simulink library "myLib_R2020a"  (R2020a)
settings: Solver=VariableStepAuto  StartTime=0.0  StopTime=10.0  RelTol=1e-3
libraries: $bdroot x26, simulink x10
settings Model: Creator=Administrator  LastModifiedBy=Administrator

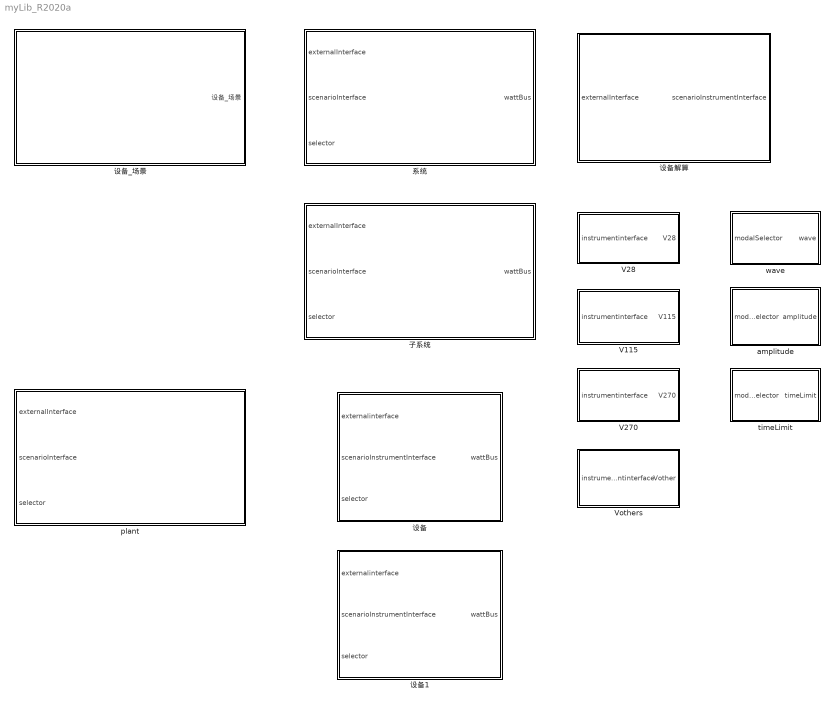
== system myLib_R2020a ==
  V115 : Subsystem  mask{V115_amplitudeData=0, V115_waveData=0, V115_timeLimitData=0}
      settings: CopyFcn=set_param(gcbh,'LinkStatus','none');
  V270 : Subsystem  mask{V270_amplitudeData=0, V270_waveData=0, V270_timeLimitData=0}
      settings: CopyFcn=set_param(gcbh,'LinkStatus','none');
  V28 : Subsystem  mask{V28_amplitudeData=0, V28_waveData=0, V28_timeLimitData=0}
      settings: CopyFcn=set_param(gcbh,'LinkStatus','none');
  Vothers : Subsystem  mask{Vother_amplitudeData=0, Vother_waveData=0, Vother_timeLimitData=0}
      settings: CopyFcn=set_param(gcbh,'LinkStatus','none');
  amplitude : Subsystem  mask{amplitudeData=[5,6,4,9,2,10]}
      settings: CopyFcn=set_param(gcbh,'LinkStatus','none');
  plant : Subsystem
      settings: CopyFcn=set_param(gcbh,'LinkStatus','none');
  timeLimit : Subsystem  mask{timeLimitData=[1 2 3 4 5 6]}
      settings: CopyFcn=set_param(gcbh,'LinkStatus','none');
  wave : Subsystem  mask{waveData=[1,2;3,4;5,6;7,8;1,2;3,4;5,6;7,8]'}
      settings: CopyFcn=set_param(gcbh,'LinkStatus','none');
      mask DialogControl ParameterGroupVar Prompt: 说明
  子系统 : Subsystem
      settings: CopyFcn=set_param(gcbh,'LinkStatus','none');
  系统 : Subsystem
      settings: CopyFcn=set_param(gcbh,'LinkStatus','none');
  设备 : Subsystem
      settings: CopyFcn=set_param(gcbh,'LinkStatus','none');
  设备1 : Subsystem
      settings: CopyFcn=set_param(gcbh,'LinkStatus','none');
  设备_场景 : Subsystem  mask{modalSelectorSig=[0 1;0 0;1 2;1 2;0 0], triggerSig=[0 1;0 0;1 0;1 0;0 0], sampleTime=-1}
      mask prompts: modalSelectorSig "模态选择信号"; triggerSig "触发信号"; sampleTime "采样时间"
  设备解算 : Subsystem

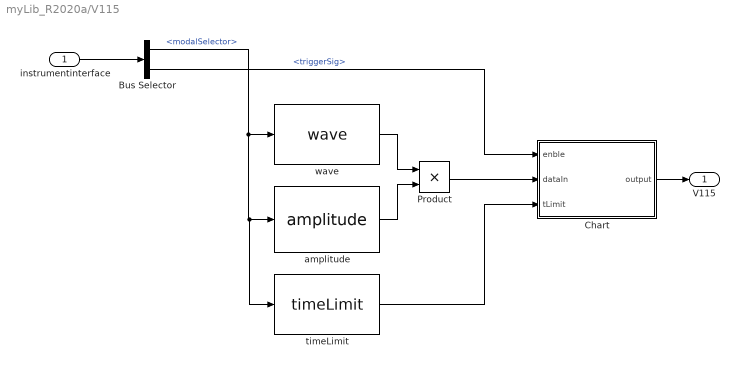
== system myLib_R2020a/V115 ==
  instrumentinterface : Inport  OutDataTypeStr=Bus: instrumentBus
  Bus Selector : BusSelector  OutputSignals=modalSelector,triggerSig
  Chart : Stateflow chart  TreatAsAtomicUnit=on
  Product : Product
  amplitude : $bdroot/amplitude  amplitudeData=V115_amplitudeData
  timeLimit : $bdroot/timeLimit  timeLimitData=V115_timeLimitData
  wave : $bdroot/wave  waveData=V115_waveData
  V115 : Outport
  wires:
  Chart/1(output) -> V115/1
  Bus Selector/1 -> wave/1, amplitude/1, timeLimit/1  "<modalSelector>"
  wave/1 -> Product/1
  Product/1 -> Chart/2(dataIn)
  amplitude/1 -> Product/2
  instrumentinterface/1 -> Bus Selector/1
  Bus Selector/2 -> Chart/1(enble)  "<triggerSig>"
  timeLimit/1 -> Chart/3(tLimit)

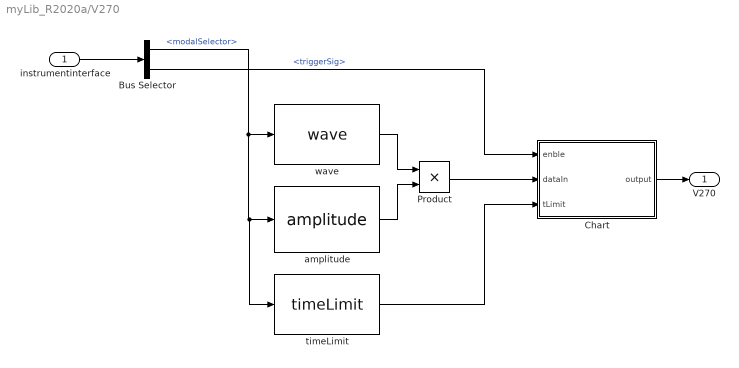
== system myLib_R2020a/V270 ==
  instrumentinterface : Inport  OutDataTypeStr=Bus: instrumentBus
  Bus Selector : BusSelector  OutputSignals=modalSelector,triggerSig
  Chart : Stateflow chart  TreatAsAtomicUnit=on
  Product : Product
  amplitude : $bdroot/amplitude  amplitudeData=V270_amplitudeData
  timeLimit : $bdroot/timeLimit  timeLimitData=V270_timeLimitData
  wave : $bdroot/wave  waveData=V270_waveData
  V270 : Outport
  wires:
  Chart/1(output) -> V270/1
  Bus Selector/1 -> timeLimit/1, amplitude/1, wave/1  "<modalSelector>"
  wave/1 -> Product/1
  Product/1 -> Chart/2(dataIn)
  amplitude/1 -> Product/2
  instrumentinterface/1 -> Bus Selector/1
  Bus Selector/2 -> Chart/1(enble)  "<triggerSig>"
  timeLimit/1 -> Chart/3(tLimit)

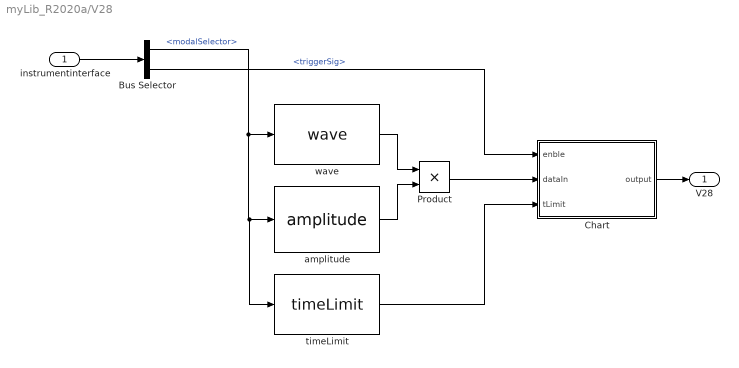
== system myLib_R2020a/V28 ==
  instrumentinterface : Inport  OutDataTypeStr=Bus: instrumentBus
  Bus Selector : BusSelector  OutputSignals=modalSelector,triggerSig
  Chart : Stateflow chart  TreatAsAtomicUnit=on
  Product : Product
  amplitude : $bdroot/amplitude  amplitudeData=V28_amplitudeData
  timeLimit : $bdroot/timeLimit  timeLimitData=V28_timeLimitData
  wave : $bdroot/wave  waveData=V28_waveData
  V28 : Outport
  wires:
  instrumentinterface/1 -> Bus Selector/1
  Bus Selector/1 -> wave/1, timeLimit/1, amplitude/1  "<modalSelector>"
  Bus Selector/2 -> Chart/1(enble)  "<triggerSig>"
  timeLimit/1 -> Chart/3(tLimit)
  wave/1 -> Product/1
  amplitude/1 -> Product/2
  Product/1 -> Chart/2(dataIn)
  Chart/1(output) -> V28/1

== system myLib_R2020a/Vothers ==
  instrumentinterface : Inport  OutDataTypeStr=Bus: instrumentBus
  Bus Selector : BusSelector  OutputSignals=modalSelector,triggerSig
  Chart : Stateflow chart  TreatAsAtomicUnit=on
  Product : Product
  amplitude : $bdroot/amplitude  amplitudeData=Vother_amplitudeData
  timeLimit : $bdroot/timeLimit  timeLimitData=Vother_timeLimitData
  wave : $bdroot/wave  waveData=Vother_waveData
  Vother : Outport
  wires:
  Chart/1(output) -> Vother/1
  Bus Selector/1 -> wave/1, amplitude/1, timeLimit/1  "<modalSelector>"
  wave/1 -> Product/1
  Product/1 -> Chart/2(dataIn)
  amplitude/1 -> Product/2
  instrumentinterface/1 -> Bus Selector/1
  Bus Selector/2 -> Chart/1(enble)  "<triggerSig>"
  timeLimit/1 -> Chart/3(tLimit)

== system myLib_R2020a/amplitude ==
  modalSelector : Inport
  Selector : Selector  IndexOptions=Starting index (port)  Indices=[1 3]  OutputSizes=1
  amplitudes : Constant  Value=amplitudeData
  amplitude : Outport
  wires:
  amplitudes/1 -> Selector/1
  modalSelector/1 -> Selector/2
  Selector/1 -> amplitude/1

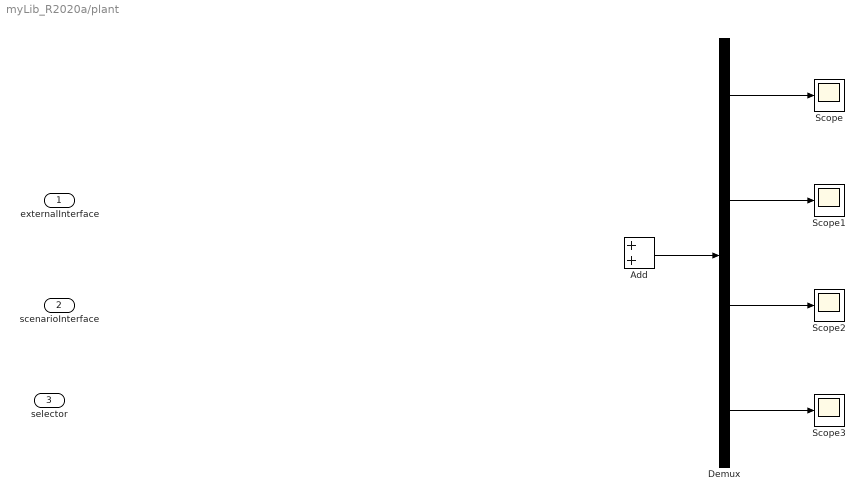
== system myLib_R2020a/plant ==
  externalInterface : Inport  OutDataTypeStr=Bus: externalBus
  scenarioInterface : Inport  Port=2  OutDataTypeStr=Bus: scenarioInstrumentBus
  selector : Inport  Port=3
  Add : Sum
  Demux : Demux
  Scope{,1..3} (4 alike) : Scope
      Scope1 settings: CopyFcn=set_param(gcbh,'LinkStatus','none');
  wires:
  Add/1 -> Demux/1
  Demux/1 -> Scope/1
  Demux/2 -> Scope1/1
  Demux/3 -> Scope2/1
  Demux/4 -> Scope3/1

== system myLib_R2020a/timeLimit ==
  modalSelector : Inport
  Selector1 : Selector  IndexOptions=Starting index (port)  Indices=[1 3]  OutputSizes=1
  timeLimits : Constant  Value=timeLimitData
  timeLimit : Outport
  wires:
  modalSelector/1 -> Selector1/2
  Selector1/1 -> timeLimit/1
  timeLimits/1 -> Selector1/1

== system myLib_R2020a/wave ==
  modalSelector : Inport
  Constant1 : Constant  Value=waveData
  Direct Lookup Table (n-D) : LookupNDDirect  InputsSelectThisObjectFromTable=Vector  TableIsInput=on  Table=[4 5 6;16 19 20;10 18 23]'
  Display : Display
  wave : Outport
  wires:
  Direct Lookup Table (n-D)/1 -> wave/1, Display/1
  Constant1/1 -> Direct Lookup Table (n-D)/2
  modalSelector/1 -> Direct Lookup Table (n-D)/1

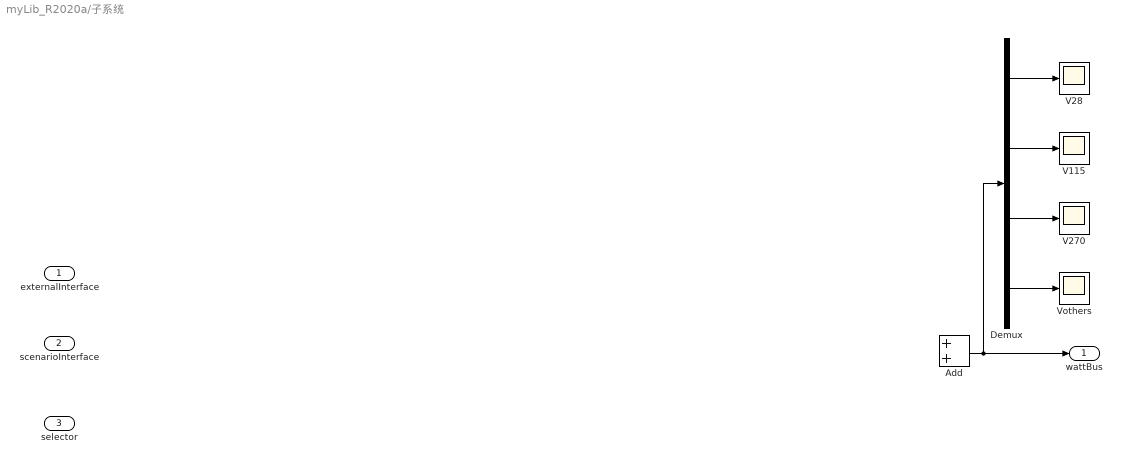
== system myLib_R2020a/子系统 ==
  externalInterface : Inport  OutDataTypeStr=Bus: externalBus
  scenarioInterface : Inport  Port=2  OutDataTypeStr=Bus: scenarioBus
  selector : Inport  Port=3
  Add : Sum
  Demux : Demux
  V115 : Scope
      settings: LoadFcn=bl = gcb
  V270 : Scope
      settings: LoadFcn=bl = gcb
  V28 : Scope
      settings: LoadFcn=bl = gcb
  Vothers : Scope
      settings: LoadFcn=bl = gcb
  wattBus : Outport  OutDataTypeStr=Bus: wattBus
  wires:
  Add/1 -> Demux/1, wattBus/1
  Demux/1 -> V28/1
  Demux/2 -> V115/1
  Demux/3 -> V270/1
  Demux/4 -> Vothers/1

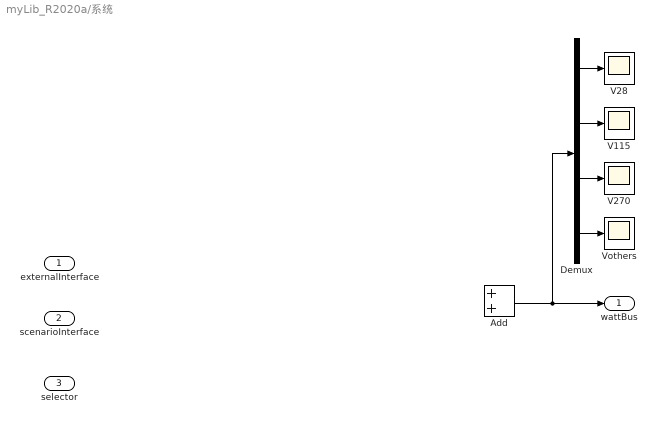
== system myLib_R2020a/系统 ==
  externalInterface : Inport  OutDataTypeStr=Bus: externalBus
  scenarioInterface : Inport  Port=2  OutDataTypeStr=Bus: scenarioBus
  selector : Inport  Port=3
  Add : Sum
  Demux : Demux
  V115 : Scope
  V270 : Scope
  V28 : Scope
  Vothers : Scope
  wattBus : Outport  OutDataTypeStr=Bus: wattBus
  wires:
  Add/1 -> Demux/1, wattBus/1
  Demux/1 -> V28/1
  Demux/2 -> V115/1
  Demux/3 -> V270/1
  Demux/4 -> Vothers/1

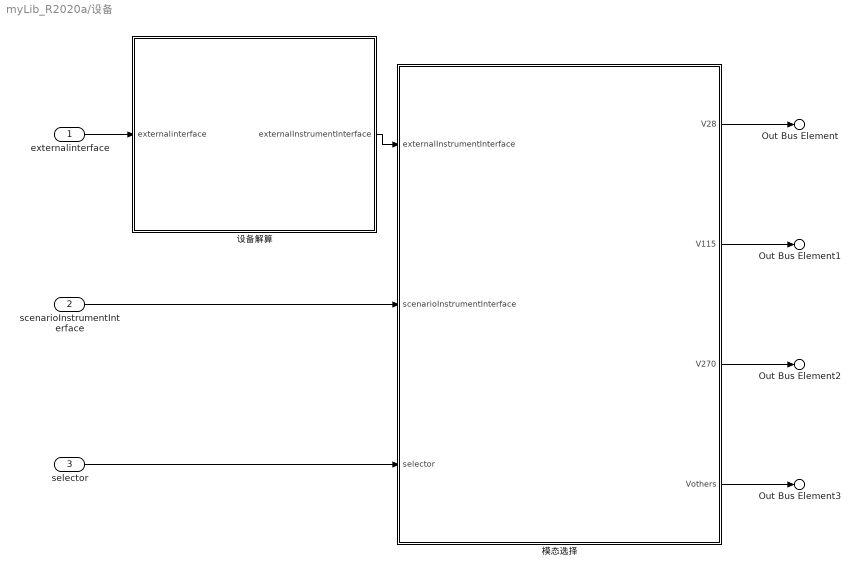
== system myLib_R2020a/设备 ==
  externalinterface : Inport  OutDataTypeStr=Bus: externalBus
  scenarioInstrumentInterface : Inport  Port=2  OutDataTypeStr=Bus: scenarioInstrumentBus
  selector : Inport  Port=3
  模态选择 : Subsystem
  设备解算 : Subsystem
  Out Bus Element : Outport  PortName=wattBus  Element=V28
  Out Bus Element1 : Outport  PortName=wattBus  Element=V115
  Out Bus Element2 : Outport  PortName=wattBus  Element=V270
  Out Bus Element3 : Outport  PortName=wattBus  Element=Vother
  wires:
  externalinterface/1 -> 设备解算/1(externalinterface)
  设备解算/1(externalInstrumentInterface) -> 模态选择/1(externalInstrumentInterface)
  scenarioInstrumentInterface/1 -> 模态选择/2(scenarioInstrumentInterface)
  模态选择/1(V28) -> Out Bus Element/1
  模态选择/2(V115) -> Out Bus Element1/1
  模态选择/3(V270) -> Out Bus Element2/1
  模态选择/4(Vothers) -> Out Bus Element3/1
  selector/1 -> 模态选择/3(selector)

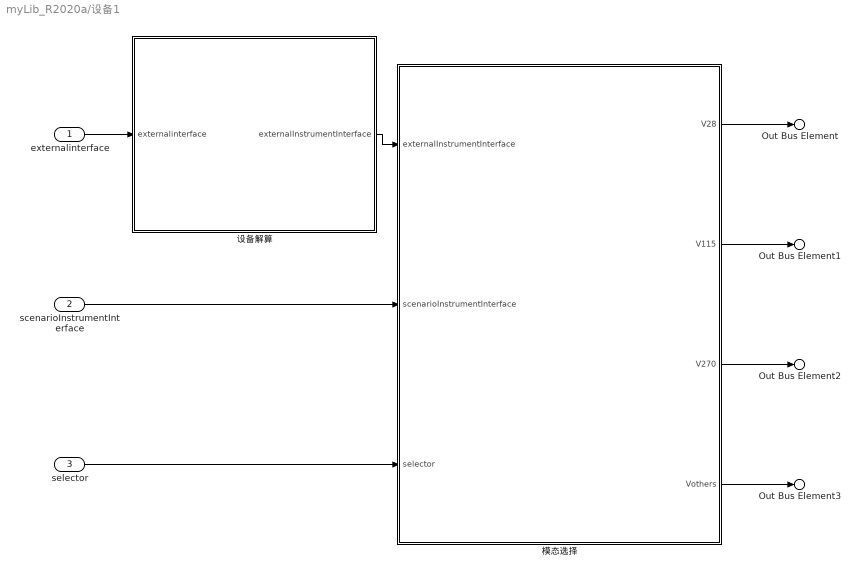
== system myLib_R2020a/设备1 ==
  externalinterface : Inport  OutDataTypeStr=Bus: externalBus
  scenarioInstrumentInterface : Inport  Port=2  OutDataTypeStr=Bus: scenarioInstrumentBus
  selector : Inport  Port=3
  模态选择 : Subsystem
  设备解算 : Subsystem
  Out Bus Element : Outport  PortName=wattBus  Element=V28
  Out Bus Element1 : Outport  PortName=wattBus  Element=V115
  Out Bus Element2 : Outport  PortName=wattBus  Element=V270
  Out Bus Element3 : Outport  PortName=wattBus  Element=Vother
  wires:
  externalinterface/1 -> 设备解算/1(externalinterface)
  设备解算/1(externalInstrumentInterface) -> 模态选择/1(externalInstrumentInterface)
  scenarioInstrumentInterface/1 -> 模态选择/2(scenarioInstrumentInterface)
  模态选择/1(V28) -> Out Bus Element/1
  模态选择/2(V115) -> Out Bus Element1/1
  模态选择/3(V270) -> Out Bus Element2/1
  模态选择/4(Vothers) -> Out Bus Element3/1
  selector/1 -> 模态选择/3(selector)

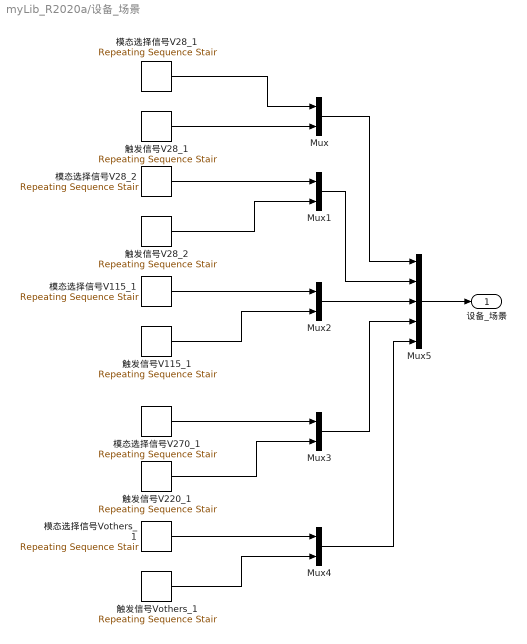
== system myLib_R2020a/设备_场景 ==
  Mux{,1..4} (5 alike) : Mux  Inputs=2
  Mux5 : Mux  Inputs=5
  模态选择信号V115_1 : simulink/Sources/Repeating Sequence Stair  OutValues=modalSelectorSig(3,:)  tsamp=sampleTime  OutMin=[]  OutMax=[]  OutDataTypeStr=double  OutputDataTypeScalingMode=double  OutDataType=fixdt(0,8)  ConRadixGroup=Best Precision: Vector-wise  OutScaling=2^-12
  模态选择信号V270_1 : simulink/Sources/Repeating Sequence Stair  OutValues=modalSelectorSig(4,:)  tsamp=sampleTime  OutMin=[]  OutMax=[]  OutDataTypeStr=double  OutputDataTypeScalingMode=double  OutDataType=fixdt(0,8)  ConRadixGroup=Best Precision: Vector-wise  OutScaling=2^-12
  模态选择信号V28_1 : simulink/Sources/Repeating Sequence Stair  OutValues=modalSelectorSig(1,:)  tsamp=sampleTime  OutMin=[]  OutMax=[]  OutDataTypeStr=double  OutputDataTypeScalingMode=double  OutDataType=fixdt(0,8)  ConRadixGroup=Best Precision: Vector-wise  OutScaling=2^-12
  模态选择信号V28_2 : simulink/Sources/Repeating Sequence Stair  OutValues=modalSelectorSig(2,:)  tsamp=sampleTime  OutMin=[]  OutMax=[]  OutDataTypeStr=double  OutputDataTypeScalingMode=double  OutDataType=fixdt(0,8)  ConRadixGroup=Best Precision: Vector-wise  OutScaling=2^-12
  模态选择信号Vothers_1 : simulink/Sources/Repeating Sequence Stair  OutValues=modalSelectorSig(5,:)  tsamp=sampleTime  OutMin=[]  OutMax=[]  OutDataTypeStr=double  OutputDataTypeScalingMode=double  OutDataType=fixdt(0,8)  ConRadixGroup=Best Precision: Vector-wise  OutScaling=2^-12
  触发信号V115_1 : simulink/Sources/Repeating Sequence Stair  OutValues=triggerSig(3,:)  tsamp=sampleTime  OutMin=[]  OutMax=[]  OutDataTypeStr=double  OutputDataTypeScalingMode=double  OutDataType=fixdt(0,8)  ConRadixGroup=Best Precision: Vector-wise  OutScaling=2^-12
  触发信号V220_1 : simulink/Sources/Repeating Sequence Stair  OutValues=triggerSig(4,:)  tsamp=sampleTime  OutMin=[]  OutMax=[]  OutDataTypeStr=double  OutputDataTypeScalingMode=double  OutDataType=fixdt(0,8)  ConRadixGroup=Best Precision: Vector-wise  OutScaling=2^-12
  触发信号V28_1 : simulink/Sources/Repeating Sequence Stair  OutValues=triggerSig(1,:)  tsamp=sampleTime  OutMin=[]  OutMax=[]  OutDataTypeStr=double  OutputDataTypeScalingMode=double  OutDataType=fixdt(0,8)  ConRadixGroup=Best Precision: Vector-wise  OutScaling=2^-12
  触发信号V28_2 : simulink/Sources/Repeating Sequence Stair  OutValues=triggerSig(2,:)  tsamp=sampleTime  OutMin=[]  OutMax=[]  OutDataTypeStr=double  OutputDataTypeScalingMode=double  OutDataType=fixdt(0,8)  ConRadixGroup=Best Precision: Vector-wise  OutScaling=2^-12
  触发信号Vothers_1 : simulink/Sources/Repeating Sequence Stair  OutValues=triggerSig(5,:)  tsamp=sampleTime  OutMin=[]  OutMax=[]  OutDataTypeStr=double  OutputDataTypeScalingMode=double  OutDataType=fixdt(0,8)  ConRadixGroup=Best Precision: Vector-wise  OutScaling=2^-12
  设备_场景 : Outport
  wires:
  模态选择信号V28_1/1 -> Mux/1
  触发信号V28_1/1 -> Mux/2
  模态选择信号V28_2/1 -> Mux1/1
  触发信号V28_2/1 -> Mux1/2
  模态选择信号V115_1/1 -> Mux2/1
  触发信号V115_1/1 -> Mux2/2
  模态选择信号V270_1/1 -> Mux3/1
  触发信号V220_1/1 -> Mux3/2
  模态选择信号Vothers_1/1 -> Mux4/1
  触发信号Vothers_1/1 -> Mux4/2
  Mux2/1 -> Mux5/3
  Mux/1 -> Mux5/1
  Mux1/1 -> Mux5/2
  Mux3/1 -> Mux5/4
  Mux4/1 -> Mux5/5
  Mux5/1 -> 设备_场景/1

== system myLib_R2020a/设备解算 ==
  externalInterface : Inport  OutDataTypeStr=Bus: externalBus
  scenarioInstrumentInterface : Outport  OutDataTypeStr=Bus: scenarioInstrumentBus

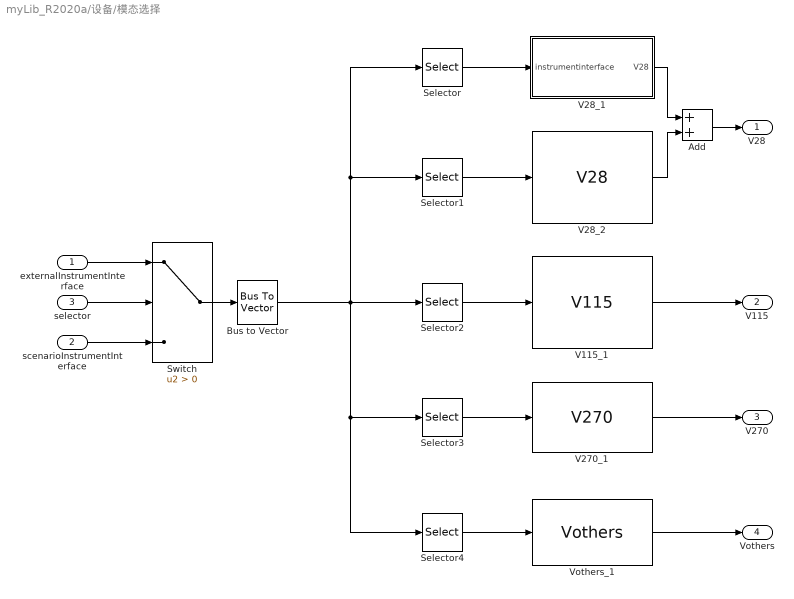
== system myLib_R2020a/设备/模态选择 ==
  externalInstrumentInterface : Inport  OutDataTypeStr=Bus: scenarioInstrumentBus
  scenarioInstrumentInterface : Inport  Port=2  OutDataTypeStr=Bus: scenarioBus
  selector : Inport  Port=3
  Add : Sum
  Bus to Vector : BusToVector
  Selector : Selector  InputPortWidth=10  IndexOptions=Index vector (dialog)  Indices=[1 6]  OutputSizes=1
  Selector1 : Selector  InputPortWidth=10  IndexOptions=Index vector (dialog)  Indices=[2 7]  OutputSizes=1
  Selector2 : Selector  InputPortWidth=10  IndexOptions=Index vector (dialog)  Indices=[3 8]  OutputSizes=1
  Selector3 : Selector  InputPortWidth=10  IndexOptions=Index vector (dialog)  Indices=[4 9]  OutputSizes=1
  Selector4 : Selector  InputPortWidth=10  IndexOptions=Index vector (dialog)  Indices=[5 10]  OutputSizes=1
  Switch : Switch  Criteria=u2 > Threshold
  V115_1 : $bdroot/V115  V115_amplitudeData=0  V115_waveData=0  V115_timeLimitData=0
  V270_1 : $bdroot/V270  V270_amplitudeData=0  V270_waveData=0  V270_timeLimitData=0
  V28_1 : Subsystem  mask{V28_amplitudeData=0, V28_waveData=0, V28_timeLimitData=0}
      settings: CopyFcn=set_param(gcbh,'LinkStatus','none');
  V28_2 : $bdroot/V28  V28_amplitudeData=0  V28_waveData=0  V28_timeLimitData=0
  Vothers_1 : $bdroot/Vothers  Vother_amplitudeData=0  Vother_waveData=0  Vother_timeLimitData=0
  V28 : Outport
  V115 : Outport  Port=2
  V270 : Outport  Port=3
  Vothers : Outport  Port=4
  wires:
  Selector1/1 -> V28_2/1
  Selector4/1 -> Vothers_1/1
  Selector2/1 -> V115_1/1
  Selector3/1 -> V270_1/1
  V270_1/1 -> V270/1
  V115_1/1 -> V115/1
  Vothers_1/1 -> Vothers/1
  selector/1 -> Switch/2
  externalInstrumentInterface/1 -> Switch/1
  scenarioInstrumentInterface/1 -> Switch/3
  Switch/1 -> Bus to Vector/1
  Selector/1 -> V28_1/1(instrumentinterface)
  Bus to Vector/1 -> Selector1/1, Selector/1, Selector4/1, Selector3/1, Selector2/1
  V28_1/1(V28) -> Add/1
  V28_2/1 -> Add/2
  Add/1 -> V28/1

== system myLib_R2020a/设备/设备解算 ==
  externalinterface : Inport  OutDataTypeStr=Bus: externalBus
  externalInstrumentInterface : Outport  OutDataTypeStr=Bus: scenarioInstrumentBus

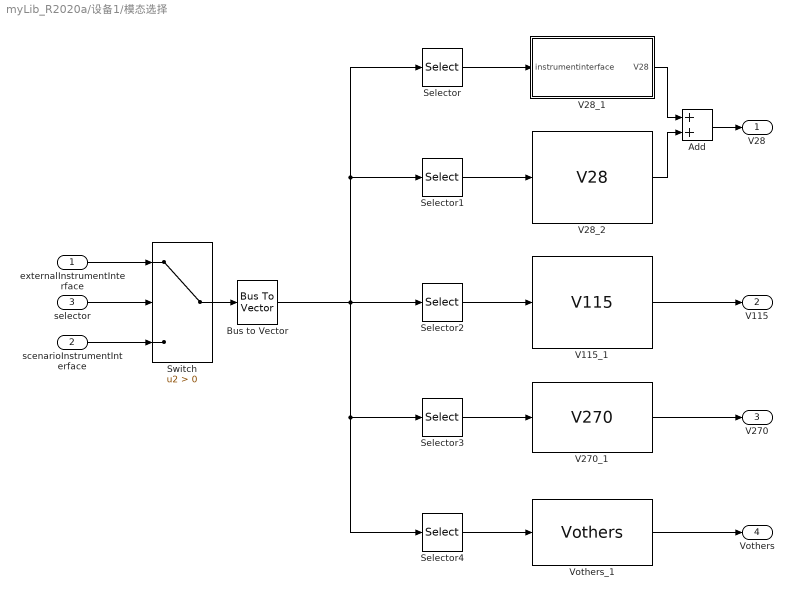
== system myLib_R2020a/设备1/模态选择 ==
  externalInstrumentInterface : Inport  OutDataTypeStr=Bus: scenarioInstrumentBus
  scenarioInstrumentInterface : Inport  Port=2  OutDataTypeStr=Bus: scenarioBus
  selector : Inport  Port=3
  Add : Sum
  Bus to Vector : BusToVector
  Selector : Selector  InputPortWidth=10  IndexOptions=Index vector (dialog)  Indices=[1 6]  OutputSizes=1
  Selector1 : Selector  InputPortWidth=10  IndexOptions=Index vector (dialog)  Indices=[2 7]  OutputSizes=1
  Selector2 : Selector  InputPortWidth=10  IndexOptions=Index vector (dialog)  Indices=[3 8]  OutputSizes=1
  Selector3 : Selector  InputPortWidth=10  IndexOptions=Index vector (dialog)  Indices=[4 9]  OutputSizes=1
  Selector4 : Selector  InputPortWidth=10  IndexOptions=Index vector (dialog)  Indices=[5 10]  OutputSizes=1
  Switch : Switch  Criteria=u2 > Threshold
  V115_1 : $bdroot/V115  V115_amplitudeData=0  V115_waveData=0  V115_timeLimitData=0
  V270_1 : $bdroot/V270  V270_amplitudeData=0  V270_waveData=0  V270_timeLimitData=0
  V28_1 : Subsystem  mask{V28_amplitudeData=0, V28_waveData=0, V28_timeLimitData=0}
      settings: CopyFcn=set_param(gcbh,'LinkStatus','none');
  V28_2 : $bdroot/V28  V28_amplitudeData=0  V28_waveData=0  V28_timeLimitData=0
  Vothers_1 : $bdroot/Vothers  Vother_amplitudeData=0  Vother_waveData=0  Vother_timeLimitData=0
  V28 : Outport
  V115 : Outport  Port=2
  V270 : Outport  Port=3
  Vothers : Outport  Port=4
  wires:
  Selector1/1 -> V28_2/1
  Selector4/1 -> Vothers_1/1
  Selector2/1 -> V115_1/1
  Selector3/1 -> V270_1/1
  V270_1/1 -> V270/1
  V115_1/1 -> V115/1
  Vothers_1/1 -> Vothers/1
  selector/1 -> Switch/2
  externalInstrumentInterface/1 -> Switch/1
  scenarioInstrumentInterface/1 -> Switch/3
  Switch/1 -> Bus to Vector/1
  Selector/1 -> V28_1/1(instrumentinterface)
  Bus to Vector/1 -> Selector1/1, Selector/1, Selector4/1, Selector3/1, Selector2/1
  V28_1/1(V28) -> Add/1
  V28_2/1 -> Add/2
  Add/1 -> V28/1

== system myLib_R2020a/设备1/设备解算 ==
  externalinterface : Inport  OutDataTypeStr=Bus: externalBus
  externalInstrumentInterface : Outport  OutDataTypeStr=Bus: scenarioInstrumentBus

== system myLib_R2020a/设备/模态选择/V28_1 ==
  instrumentinterface : Inport  OutDataTypeStr=Bus: instrumentBus
  Bus Selector : BusSelector  OutputSignals=modalSelector,triggerSig
  Chart : Stateflow chart  TreatAsAtomicUnit=on
  Product : Product
  amplitude : $bdroot/amplitude  amplitudeData=V28_amplitudeData
  timeLimit : $bdroot/timeLimit  timeLimitData=V28_timeLimitData
  wave : $bdroot/wave  waveData=V28_waveData
  V28 : Outport
  wires:
  instrumentinterface/1 -> Bus Selector/1
  Bus Selector/1 -> wave/1, timeLimit/1, amplitude/1  "<modalSelector>"
  Bus Selector/2 -> Chart/1(enble)  "<triggerSig>"
  timeLimit/1 -> Chart/3(tLimit)
  wave/1 -> Product/1
  amplitude/1 -> Product/2
  Product/1 -> Chart/2(dataIn)
  Chart/1(output) -> V28/1

== system myLib_R2020a/设备1/模态选择/V28_1 ==
  instrumentinterface : Inport  OutDataTypeStr=Bus: instrumentBus
  Bus Selector : BusSelector  OutputSignals=modalSelector,triggerSig
  Chart : Stateflow chart  TreatAsAtomicUnit=on
  Product : Product
  amplitude : $bdroot/amplitude  amplitudeData=V28_amplitudeData
  timeLimit : $bdroot/timeLimit  timeLimitData=V28_timeLimitData
  wave : $bdroot/wave  waveData=V28_waveData
  V28 : Outport
  wires:
  instrumentinterface/1 -> Bus Selector/1
  Bus Selector/1 -> wave/1, timeLimit/1, amplitude/1  "<modalSelector>"
  Bus Selector/2 -> Chart/1(enble)  "<triggerSig>"
  timeLimit/1 -> Chart/3(tLimit)
  wave/1 -> Product/1
  amplitude/1 -> Product/2
  Product/1 -> Chart/2(dataIn)
  Chart/1(output) -> V28/1

== stateflow chart myLib_R2020a/V115/Chart ==
  state idle
    en:
    cnt=1;
  state outputs
    en:
    output=dataIn(cnt);
    cnt=cnt+1;
    du:
    output=dataIn(cnt);
    cnt=cnt+1;
    ex:
    output=0;
  (default) -> idle
  idle -> outputs : [enble]
  outputs -> idle : [cnt>=tLimit]
  data: enble input; dataIn input; tLimit input; cnt local; output output

== stateflow chart myLib_R2020a/V270/Chart ==
  state idle
    en:
    cnt=1;
  state outputs
    en:
    output=dataIn(cnt);
    cnt=cnt+1;
    du:
    output=dataIn(cnt);
    cnt=cnt+1;
    ex:
    output=0;
  (default) -> idle
  idle -> outputs : [enble]
  outputs -> idle : [cnt>=tLimit]
  data: enble input; dataIn input; tLimit input; cnt local; output output

== stateflow chart myLib_R2020a/V28/Chart ==
  state idle
    en:
    cnt=1;
  state outputs
    en:
    output=dataIn(cnt);
    cnt=cnt+1;
    du:
    output=dataIn(cnt);
    cnt=cnt+1;
    ex:
    output=0;
  (default) -> idle
  idle -> outputs : [enble]
  outputs -> idle : [cnt>=tLimit]
  data: enble input; dataIn input; tLimit input; cnt local; output output

== stateflow chart myLib_R2020a/Vothers/Chart ==
  state idle
    en:
    cnt=1;
  state outputs
    en:
    output=dataIn(cnt);
    cnt=cnt+1;
    du:
    output=dataIn(cnt);
    cnt=cnt+1;
    ex:
    output=0;
  (default) -> idle
  idle -> outputs : [enble]
  outputs -> idle : [cnt>=tLimit]
  data: enble input; dataIn input; tLimit input; cnt local; output output

== stateflow chart myLib_R2020a/设备/模态选择/V28_1/Chart ==
  state idle
    en:
    cnt=1;
  state outputs
    en:
    output=dataIn(cnt);
    cnt=cnt+1;
    du:
    output=dataIn(cnt);
    cnt=cnt+1;
    ex:
    output=0;
  (default) -> idle
  idle -> outputs : [enble]
  outputs -> idle : [cnt>=tLimit]
  data: enble input; dataIn input; tLimit input; cnt local; output output

== stateflow chart myLib_R2020a/设备1/模态选择/V28_1/Chart ==
  state idle
    en:
    cnt=1;
  state outputs
    en:
    output=dataIn(cnt);
    cnt=cnt+1;
    du:
    output=dataIn(cnt);
    cnt=cnt+1;
    ex:
    output=0;
  (default) -> idle
  idle -> outputs : [enble]
  outputs -> idle : [cnt>=tLimit]
  data: enble input; dataIn input; tLimit input; cnt local; output output
